simulink model "firmwareV1000_flight_replay"  (R2020b)
settings: Solver=ode1  StartTime=tspan(1)  StopTime=tspan(2)  FixedStep=Ts_SimBigModel.Ts_base  RelTol=1e-3
settings Model: PauseTimes=1  Creator=sl  LastModifiedBy=sl
settings SolverCC: AutoInsertRateTranBlk=on
settings OptimizationCC: DefaultParameterBehavior=Inlined  EnhancedBackFolding=on  PassReuseOutputArgsAs=Individual arguments  ZeroExternalMemoryAtStartup=off  ZeroInternalMemoryAtStartup=off  MaxStackSize=64  OptimizeBlockOrder=speed  DifferentSizesBufferReuse=on  OptimizationCustomize=off  EfficientTunableParamExpr=on
settings DebuggingCC: InheritedTsInSrcMsg=none  MultiTaskCondExecSysMsg=none  ParameterTunabilityLossMsg=error  UnconnectedInputMsg=none  UnconnectedOutputMsg=none  UnconnectedLineMsg=none  BusObjectLabelMismatch=error  SFUnusedDataAndEventsDiag=none
settings HardwareCC: ProdBitPerPointer=32  ProdBitPerSizeT=32  ProdBitPerPtrDiffT=32  ProdLargestAtomicInteger=Long  ProdLargestAtomicFloat=Double  ProdWordSize=32  ProdHWDeviceType=ARM Compatible->ARM Cortex
settings ModelReferenceCC: EnableParallelModelReferenceBuilds=on  ParallelModelReferenceMATLABWorkerInit=Load Top Model
settings SFSimCC: MATLABDynamicMemAlloc=off
settings RTWCC: Description=Embedded Coder  SystemTargetFile=ert.tlc  TemplateMakefile=ert_default_tmf  GenerateReport=on  Toolchain=Microsoft Visual C++ 2017 v15.0 | nmake (64-bit Windows)  IncludeHyperlinkInReport=on  LaunchReport=on  GenerateTraceInfo=on  GenerateTraceReport=on  GenerateTraceReportSl=on  GenerateTraceReportSf=on  GenerateTraceReportEml=on
settings CodeAppCC: ForceParamTrailComments=on  IgnoreCustomStorageClasses=off  OperatorAnnotations=on  SimulinkDataObjDesc=on  SFDataObjDesc=on  InsertBlockDesc=on
settings ERTTargetCC: InlinedParameterPlacement=NonHierarchical  ERTCustomFileTemplate=example_file_process.tlc

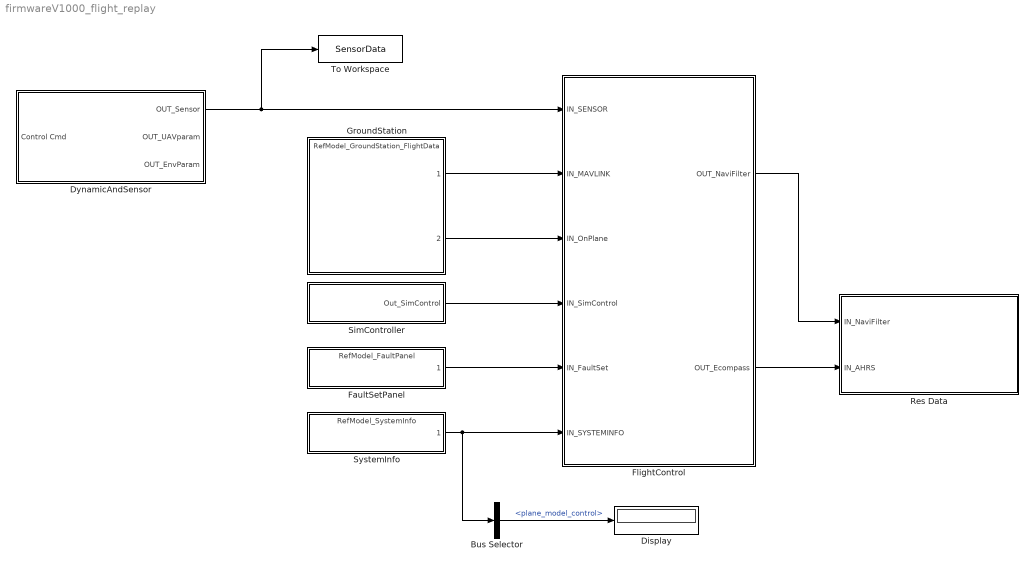
== system firmwareV1000_flight_replay ==
  Bus Selector : BusSelector  OutputSignals=plane_model_control
  Display : Display
  DynamicAndSensor : Subsystem  Variant=on
  FaultSetPanel : ModelReference  ModelNameDialog=RefModel_FaultPanel  SimulationMode=Normal  ModelReferenceVersion=2.3
  FlightControl : Subsystem
  GroundStation : ModelReference  ModelNameDialog=RefModel_GroundStation_FlightData.slx  SimulationMode=Normal  CachedPortDiscreteRates=[0.04]  ModelReferenceVersion=2.13
  Res Data : Subsystem
  SimController : Subsystem  VariantControl=SensorNoiseMode==1
  SystemInfo : ModelReference  ModelNameDialog=RefModel_SystemInfo.slx  SimulationMode=Normal  ModelReferenceVersion=2.14
  To Workspace : ToWorkspace  VariableName=SensorData  SaveFormat=Timeseries  SampleTime=-1
  wires:
  DynamicAndSensor/1(OUT_Sensor) -> FlightControl/1(IN_SENSOR), To Workspace/1
  GroundStation/2 -> FlightControl/3(IN_OnPlane)
  GroundStation/1 -> FlightControl/2(IN_MAVLINK)
  SimController/1(Out_SimControl) -> FlightControl/4(IN_SimControl)
  FaultSetPanel/1 -> FlightControl/5(IN_FaultSet)
  FlightControl/1(OUT_NaviFilter) -> Res Data/1(IN_NaviFilter)
  SystemInfo/1 -> Bus Selector/1, FlightControl/6(IN_SYSTEMINFO)
  Bus Selector/1 -> Display/1  "<plane_model_control>"
  FlightControl/2(OUT_Ecompass) -> Res Data/2(IN_AHRS)

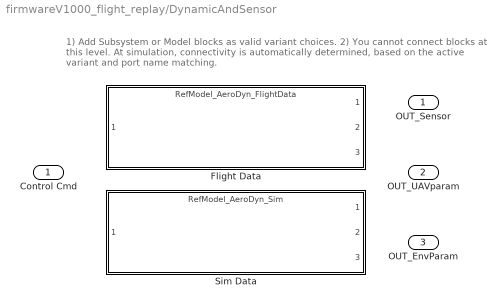
== system firmwareV1000_flight_replay/DynamicAndSensor ==
  note: 1) Add Subsystem or Model blocks as valid variant choices.
      | 2) You cannot connect blocks at this level. At simulation, connectivity is automatically
      | determined, based on the active variant and port name matching.
  Control Cmd : Inport  OutDataTypeStr=Bus: BUS_CONTROL_ACTUATOR
  Flight Data : ModelReference  DisableCoverage=on  ModelNameDialog=RefModel_AeroDyn_FlightData.slx  SimulationMode=Normal  VariantControl=SimulinkRunMode == 1  ModelReferenceVersion=2.72
  Sim Data : ModelReference  ModelNameDialog=RefModel_AeroDyn_Sim.slx  SimulationMode=Normal  VariantControl=SimulinkRunMode == 2  ModelReferenceVersion=3.4
  OUT_Sensor : Outport
  OUT_UAVparam : Outport  Port=2
  OUT_EnvParam : Outport  Port=3  LockScale=on

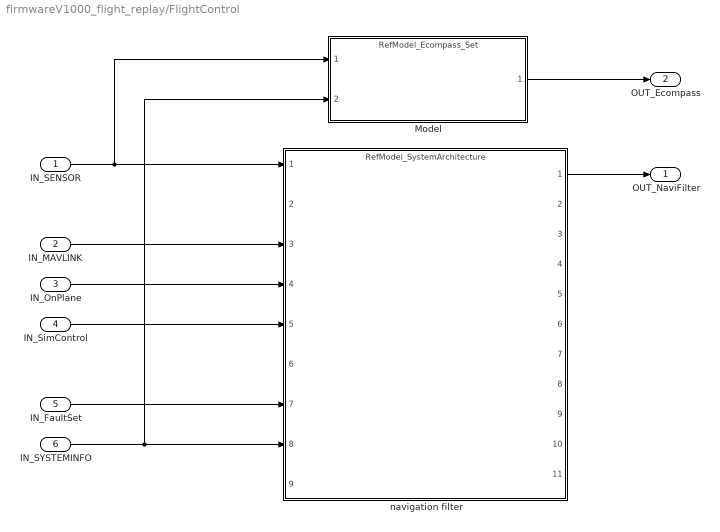
== system firmwareV1000_flight_replay/FlightControl ==
  IN_SENSOR : Inport
  IN_MAVLINK : Inport  Port=2
  IN_OnPlane : Inport  Port=3
  IN_SimControl : Inport  Port=4
  IN_FaultSet : Inport  Port=5
  IN_SYSTEMINFO : Inport  Port=6
  Model : ModelReference  ModelNameDialog=RefModel_Ecompass_Set.slx  SimulationMode=Normal  ModelReferenceVersion=2.178
  navigation filter : ModelReference  ModelNameDialog=RefModel_SystemArchitecture  SimulationMode=Normal  ModelReferenceVersion=2.174
  OUT_NaviFilter : Outport
  OUT_Ecompass : Outport  Port=2
  wires:
  IN_MAVLINK/1 -> navigation filter/3
  IN_OnPlane/1 -> navigation filter/4
  IN_SimControl/1 -> navigation filter/5
  IN_FaultSet/1 -> navigation filter/7
  navigation filter/1 -> OUT_NaviFilter/1
  IN_SENSOR/1 -> Model/1, navigation filter/1
  IN_SYSTEMINFO/1 -> Model/2, navigation filter/8
  Model/1 -> OUT_Ecompass/1

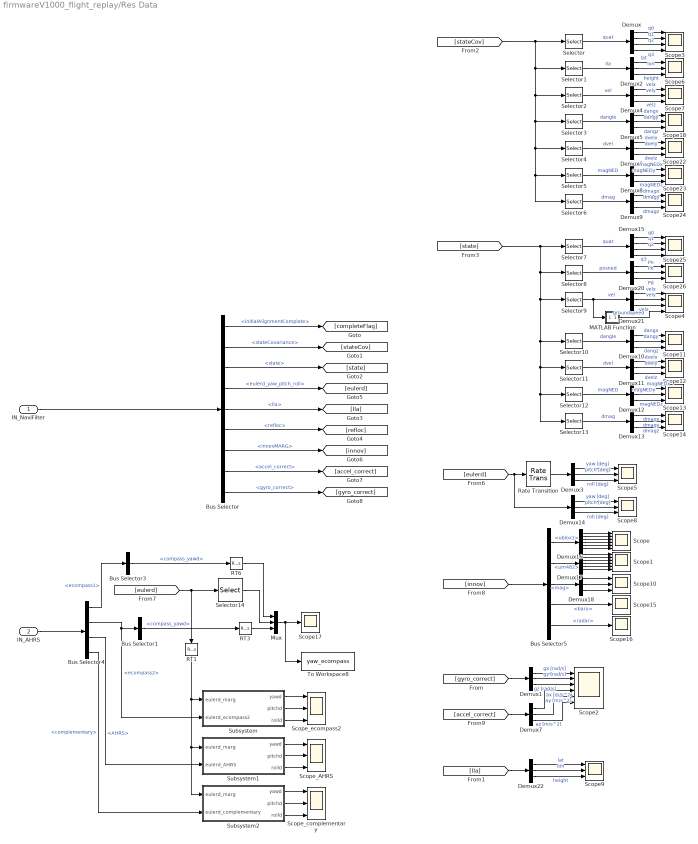
== system firmwareV1000_flight_replay/Res Data ==
  IN_NaviFilter : Inport
  IN_AHRS : Inport  Port=2
  Bus Selector : BusSelector  OutputSignals=Status.initialAlignmentComplete,stateCovariance,state,eulerd_yaw_pitch_roll,lla,InitValue.refloc,innovMARG,accel_correct,gyro_correct
  Bus Selector1 : BusSelector  OutputSignals=compass_yawd
  Bus Selector3 : BusSelector  OutputSignals=compass_yawd
  Bus Selector4 : BusSelector  OutputSignals=ecompass1,ecompass2,AHRS,complementary
  Bus Selector5 : BusSelector  OutputSignals=ublox1,um482,mag,baro,radar
  Demux : Demux
  Demux{1..14,18,20..22} (18 alike) : Demux  Outputs=3
  Demux15 : Demux
  Demux16 : Demux  Outputs=6
  Demux17 : Demux  Outputs=6
  MATLAB Function : MATLAB Function  TreatAsAtomicUnit=on
  Mux : Mux  Inputs=3
  RT1 : RateTransition
  RT3 : RateTransition
  RT6 : RateTransition
  Rate Transition : RateTransition
  Scope : Scope  NumInputPorts=6
  Scope1 : Scope  NumInputPorts=6
  Scope{5..14,18,22..24,26} (15 alike) : Scope  NumInputPorts=3
  Scope15 : Scope
  Scope16 : Scope
  Scope17 : Scope
  Scope2 : Scope  NumInputPorts=6
  Scope25 : Scope  NumInputPorts=4
  Scope3 : Scope  NumInputPorts=4
  Scope4 : Scope  NumInputPorts=4
  Scope_AHRS : Scope  NumInputPorts=3
  Scope_complementary : Scope  NumInputPorts=3
  Scope_ecompass2 : Scope  NumInputPorts=3
  Selector : Selector  InputPortWidth=NAVI_PARAM_BASE.nStateMARG24  IndexOptions=Index vector (dialog)  Indices=[1:4]  OutputSizes=1
  Selector1 : Selector  InputPortWidth=NAVI_PARAM_BASE.nStateMARG24  IndexOptions=Index vector (dialog)  Indices=[5:7]  OutputSizes=1
  Selector10 : Selector  InputPortWidth=NAVI_PARAM_BASE.nStateMARG24  IndexOptions=Index vector (dialog)  Indices=[11:13]  OutputSizes=1
  Selector11 : Selector  InputPortWidth=NAVI_PARAM_BASE.nStateMARG24  IndexOptions=Index vector (dialog)  Indices=[14:16]  OutputSizes=1
  Selector12 : Selector  InputPortWidth=NAVI_PARAM_BASE.nStateMARG24  IndexOptions=Index vector (dialog)  Indices=[17:19]  OutputSizes=1
  Selector13 : Selector  InputPortWidth=NAVI_PARAM_BASE.nStateMARG24  IndexOptions=Index vector (dialog)  Indices=[20:22]  OutputSizes=1
  Selector14 : Selector  InputPortWidth=3  IndexOptions=Index vector (dialog)  Indices=1  OutputSizes=1
  Selector2 : Selector  InputPortWidth=NAVI_PARAM_BASE.nStateMARG24  IndexOptions=Index vector (dialog)  Indices=[8:10]  OutputSizes=1
  Selector3 : Selector  InputPortWidth=NAVI_PARAM_BASE.nStateMARG24  IndexOptions=Index vector (dialog)  Indices=[11:13]  OutputSizes=1
  Selector4 : Selector  InputPortWidth=NAVI_PARAM_BASE.nStateMARG24  IndexOptions=Index vector (dialog)  Indices=[14:16]  OutputSizes=1
  Selector5 : Selector  InputPortWidth=NAVI_PARAM_BASE.nStateMARG24  IndexOptions=Index vector (dialog)  Indices=[17:19]  OutputSizes=1
  Selector6 : Selector  InputPortWidth=NAVI_PARAM_BASE.nStateMARG24  IndexOptions=Index vector (dialog)  Indices=[20:22]  OutputSizes=1
  Selector7 : Selector  InputPortWidth=NAVI_PARAM_BASE.nStateMARG24  IndexOptions=Index vector (dialog)  Indices=[1:4]  OutputSizes=1
  Selector8 : Selector  InputPortWidth=NAVI_PARAM_BASE.nStateMARG24  IndexOptions=Index vector (dialog)  Indices=[5:7]  OutputSizes=1
  Selector9 : Selector  InputPortWidth=NAVI_PARAM_BASE.nStateMARG24  IndexOptions=Index vector (dialog)  Indices=[8:10]  OutputSizes=1
  Subsystem : Subsystem
  Subsystem1 : Subsystem
  Subsystem2 : Subsystem
  To Workspace8 : ToWorkspace  VariableName=yaw_ecompass  SaveFormat=Timeseries  SampleTime=-1
  wires:
  Demux13/1 -> Scope14/1  "dmagx"
  Demux12/2 -> Scope13/2  "magNEDy"
  Demux12/1 -> Scope13/1  "magNEDx"
  Demux3/2 -> Scope5/2  "pitch [deg]"
  Selector10/1 -> Demux10/1  "dangle"
  Demux21/3 -> Scope4/3  "velz"
  Selector14/1 -> Mux/2
  Demux/2 -> Scope3/2  "q1"
  [eulerd] -> Selector14/1, RT1/1
  [state] -> Selector8/1, Selector11/1, Selector12/1, Selector13/1, Selector10/1, Selector9/1, Selector7/1
  Demux6/3 -> Scope22/3  "dvelz"
  Demux5/2 -> Scope18/2  "dangy"
  Demux11/1 -> Scope12/1  "dvelx"
  Bus Selector1/1 -> RT3/1  "<compass_yawd>"
  Subsystem/3(rolld) -> Scope_ecompass2/3
  Demux16/3 -> Scope/3
  Demux3/1 -> Scope5/1  "yaw [deg]"
  Bus Selector5/5 -> Scope16/1  "<radar>"
  Demux17/1 -> Scope1/1
  Bus Selector4/1 -> Bus Selector3/1  "<ecompass1>"
  Bus Selector5/4 -> Scope15/1  "<baro>"
  Demux/1 -> Scope3/1  "q0"
  Demux6/2 -> Scope22/2  "dvely"
  Demux9/1 -> Scope24/1  "dmagx"
  Bus Selector/9 -> [gyro_correct]  "<gyro_correct>"
  Bus Selector5/2 -> Demux17/1  "<um482>"
  Demux2/3 -> Scope6/3  "height"
  Demux14/3 -> Scope8/3  "roll [deg]"
  RT1/1 -> Subsystem2/1(eulerd_marg), Subsystem1/1(eulerd_marg), Subsystem/1(eulerd_marg)
  Selector1/1 -> Demux2/1  "lla"
  Demux18/1 -> Scope10/1
  Demux21/2 -> Scope4/2  "vely"
  Bus Selector4/4 -> Subsystem2/2(eulerd_complementary)  "<complementary>"
  Bus Selector5/3 -> Demux18/1  "<mag>"
  Demux17/2 -> Scope1/2
  [lla] -> Demux22/1
  Rate Transition/1 -> Demux3/1
  Bus Selector/4 -> [eulerd]  "<eulerd_yaw_pitch_roll>"
  Subsystem1/1(yawd) -> Scope_AHRS/1
  Demux6/1 -> Scope22/1  "dvelx"
  Demux17/4 -> Scope1/4
  Demux17/3 -> Scope1/3
  Demux11/2 -> Scope12/2  "dvely"
  Bus Selector5/1 -> Demux16/1  "<ublox1>"
  Demux16/1 -> Scope/1
  MATLAB Function/1(y) -> Scope4/4  "groundspeed"
  Demux20/1 -> Scope26/1  "Pn"
  Demux17/6 -> Scope1/6
  Demux16/4 -> Scope/4
  Demux15/2 -> Scope25/2  "q1"
  Demux16/5 -> Scope/5
  Bus Selector4/2 -> Subsystem/2(eulerd_ecompass2), Bus Selector1/1  "<ecompass2>"
  Demux17/5 -> Scope1/5
  Bus Selector/2 -> [stateCov]  "<stateCovariance>"
  Demux10/1 -> Scope11/1  "dangx"
  Selector12/1 -> Demux12/1  "magNED"
  IN_NaviFilter/1 -> Bus Selector/1
  Demux4/3 -> Scope7/3  "velz"
  Mux/1 -> To Workspace8/1, Scope17/1
  [eulerd] -> Demux14/1, Rate Transition/1
  Subsystem/2(pitchd) -> Scope_ecompass2/2
  Bus Selector/5 -> [lla]  "<lla>"
  Subsystem1/3(rolld) -> Scope_AHRS/3
  Demux14/1 -> Scope8/1  "yaw [deg]"
  Subsystem2/3(rolld) -> Scope_complementary/3
  Subsystem2/1(yawd) -> Scope_complementary/1
  Selector2/1 -> Demux4/1  "vel"
  Demux3/3 -> Scope5/3  "roll [deg]"
  Subsystem2/2(pitchd) -> Scope_complementary/2
  Subsystem/1(yawd) -> Scope_ecompass2/1
  Demux1/2 -> Scope2/2  "gy [rad/s]"
  Demux22/3 -> Scope9/3  "height"
  Demux22/1 -> Scope9/1  "lat"
  Demux15/3 -> Scope25/3  "q2"
  Demux1/3 -> Scope2/3  "gz [rad/s]"
  Selector5/1 -> Demux8/1  "magNED"
  Bus Selector3/1 -> RT6/1  "<compass_yawd>"
  Demux7/1 -> Scope2/4  "ax [m/s^2]"
  Demux1/1 -> Scope2/1  "gx [rad/s]"
  Bus Selector/7 -> [innov]  "<innovMARG>"
  Demux14/2 -> Scope8/2  "pitch [deg]"
  [innov] -> Bus Selector5/1
  [accel_correct] -> Demux7/1
  Demux7/3 -> Scope2/6  "az [m/s^2]"
  Bus Selector/3 -> [state]  "<state>"
  Demux11/3 -> Scope12/3  "dvelz"
  Demux5/3 -> Scope18/3  "dangz"
  Bus Selector/1 -> [completeFlag]  "<initialAlignmentComplete>"
  Bus Selector/8 -> [accel_correct]  "<accel_correct>"
  Bus Selector/6 -> [refloc]  "<refloc>"
  Demux20/3 -> Scope26/3  "Pd"
  Demux8/3 -> Scope23/3  "magNEDz"
  Demux4/1 -> Scope7/1  "velx"
  Demux5/1 -> Scope18/1  "dangx"
  Selector4/1 -> Demux6/1  "dvel"
  Demux9/2 -> Scope24/2  "dmagy"
  Demux10/2 -> Scope11/2  "dangy"
  [gyro_correct] -> Demux1/1
  Demux2/2 -> Scope6/2  "lon"
  Demux10/3 -> Scope11/3  "dangz"
  Demux16/2 -> Scope/2
  Selector11/1 -> Demux11/1  "dvel"
  Demux13/3 -> Scope14/3  "dmagz"
  Demux18/2 -> Scope10/2
  Selector8/1 -> Demux20/1  "posned"
  Demux4/2 -> Scope7/2  "vely"
  Demux13/2 -> Scope14/2  "dmagy"
  Selector9/1 -> MATLAB Function/1(vel), Demux21/1  "vel"
  Subsystem1/2(pitchd) -> Scope_AHRS/2
  Demux12/3 -> Scope13/3  "magNEDz"
  Selector7/1 -> Demux15/1  "quat"
  Demux8/2 -> Scope23/2  "magNEDy"
  Demux/3 -> Scope3/3  "q2"
  Demux15/4 -> Scope25/4  "q3"
  Bus Selector4/3 -> Subsystem1/2(eulerd_AHRS)  "<AHRS>"
  IN_AHRS/1 -> Bus Selector4/1
  Selector13/1 -> Demux13/1  "dmag"
  Demux8/1 -> Scope23/1  "magNEDx"
  Demux21/1 -> Scope4/1  "velx"
  Demux9/3 -> Scope24/3  "dmagz"
  Selector3/1 -> Demux5/1  "dangle"
  Demux18/3 -> Scope10/3
  Demux/4 -> Scope3/4  "q3"
  RT3/1 -> Mux/3
  Selector6/1 -> Demux9/1  "dmag"
  Demux20/2 -> Scope26/2  "Pe"
  Demux7/2 -> Scope2/5  "ay [m/s^2]"
  Demux22/2 -> Scope9/2  "lon"
  Demux15/1 -> Scope25/1  "q0"
  [stateCov] -> Selector/1, Selector3/1, Selector4/1, Selector5/1, Selector6/1, Selector2/1, Selector1/1
  Demux2/1 -> Scope6/1  "lat"
  Demux16/6 -> Scope/6
  Selector/1 -> Demux/1  "quat"
  RT6/1 -> Mux/1

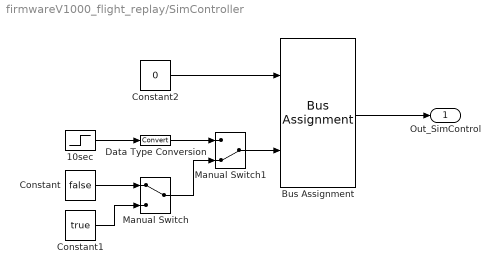
== system firmwareV1000_flight_replay/SimController ==
  10sec : Step  Time=10+33  mask(DiscretizedSource){}
      mask init:
      | %zoh
  Bus Assignment : BusAssignment  AssignedSignals=isSimOn
  Constant : Constant  Value=false
  Constant1 : Constant  Value=true
  Constant2 : Constant  Value=0  OutDataTypeStr=Bus: BUS_SIMCONTROL
  Data Type Conversion : DataTypeConversion
  Manual Switch : ManualSwitch
  Manual Switch1 : ManualSwitch  CurrentSetting=0
  Out_SimControl : Outport
  wires:
  Constant/1 -> Manual Switch/1
  Constant1/1 -> Manual Switch/2
  Constant2/1 -> Bus Assignment/1
  Bus Assignment/1 -> Out_SimControl/1
  Manual Switch1/1 -> Bus Assignment/2
  Manual Switch/1 -> Manual Switch1/2
  10sec/1 -> Data Type Conversion/1
  Data Type Conversion/1 -> Manual Switch1/1

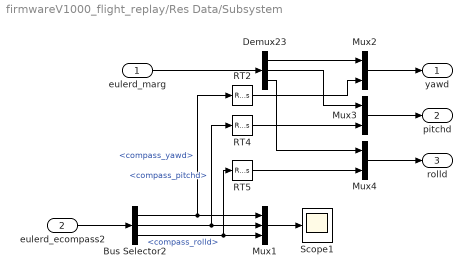
== system firmwareV1000_flight_replay/Res Data/Subsystem ==
  eulerd_marg : Inport
  eulerd_ecompass2 : Inport  Port=2
  Bus Selector2 : BusSelector  OutputSignals=compass_yawd,compass_pitchd,compass_rolld
  Demux23 : Demux  Outputs=3
  Mux1 : Mux  Inputs=3
  Mux2 : Mux  Inputs=2
  Mux3 : Mux  Inputs=2
  Mux4 : Mux  Inputs=2
  RT2 : RateTransition
  RT4 : RateTransition
  RT5 : RateTransition
  Scope1 : Scope
  yawd : Outport
  pitchd : Outport  Port=2
  rolld : Outport  Port=3
  wires:
  RT4/1 -> Mux3/2
  Demux23/1 -> Mux2/1
  RT2/1 -> Mux2/2
  Mux1/1 -> Scope1/1
  Bus Selector2/2 -> RT4/1, Mux1/2  "<compass_pitchd>"
  Demux23/3 -> Mux4/1
  eulerd_marg/1 -> Demux23/1
  Bus Selector2/3 -> RT5/1, Mux1/3  "<compass_rolld>"
  RT5/1 -> Mux4/2
  Demux23/2 -> Mux3/1
  Bus Selector2/1 -> Mux1/1, RT2/1  "<compass_yawd>"
  Mux4/1 -> rolld/1
  eulerd_ecompass2/1 -> Bus Selector2/1
  Mux3/1 -> pitchd/1
  Mux2/1 -> yawd/1

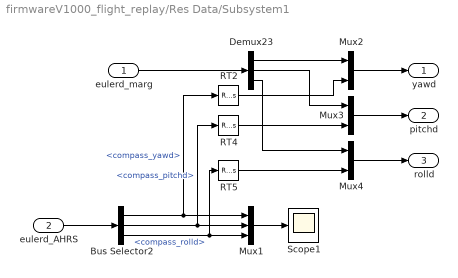
== system firmwareV1000_flight_replay/Res Data/Subsystem1 ==
  eulerd_marg : Inport
  eulerd_AHRS : Inport  Port=2
  Bus Selector2 : BusSelector  OutputSignals=compass_yawd,compass_pitchd,compass_rolld
  Demux23 : Demux  Outputs=3
  Mux1 : Mux  Inputs=3
  Mux2 : Mux  Inputs=2
  Mux3 : Mux  Inputs=2
  Mux4 : Mux  Inputs=2
  RT2 : RateTransition
  RT4 : RateTransition
  RT5 : RateTransition
  Scope1 : Scope
  yawd : Outport
  pitchd : Outport  Port=2
  rolld : Outport  Port=3
  wires:
  Mux2/1 -> yawd/1
  Mux3/1 -> pitchd/1
  eulerd_AHRS/1 -> Bus Selector2/1
  Mux4/1 -> rolld/1
  Bus Selector2/1 -> RT2/1, Mux1/1  "<compass_yawd>"
  Demux23/2 -> Mux3/1
  RT5/1 -> Mux4/2
  Bus Selector2/3 -> Mux1/3, RT5/1  "<compass_rolld>"
  eulerd_marg/1 -> Demux23/1
  Demux23/3 -> Mux4/1
  Bus Selector2/2 -> Mux1/2, RT4/1  "<compass_pitchd>"
  Mux1/1 -> Scope1/1
  RT2/1 -> Mux2/2
  Demux23/1 -> Mux2/1
  RT4/1 -> Mux3/2

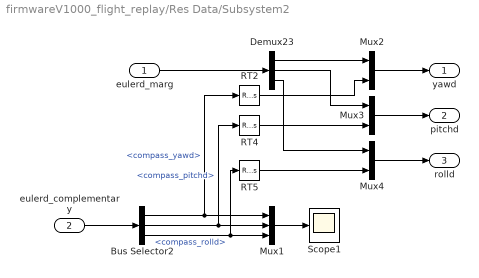
== system firmwareV1000_flight_replay/Res Data/Subsystem2 ==
  eulerd_marg : Inport
  eulerd_complementary : Inport  Port=2
  Bus Selector2 : BusSelector  OutputSignals=compass_yawd,compass_pitchd,compass_rolld
  Demux23 : Demux  Outputs=3
  Mux1 : Mux  Inputs=3
  Mux2 : Mux  Inputs=2
  Mux3 : Mux  Inputs=2
  Mux4 : Mux  Inputs=2
  RT2 : RateTransition
  RT4 : RateTransition
  RT5 : RateTransition
  Scope1 : Scope
  yawd : Outport
  pitchd : Outport  Port=2
  rolld : Outport  Port=3
  wires:
  RT4/1 -> Mux3/2
  Demux23/1 -> Mux2/1
  RT2/1 -> Mux2/2
  Mux1/1 -> Scope1/1
  Bus Selector2/2 -> RT4/1, Mux1/2  "<compass_pitchd>"
  Demux23/3 -> Mux4/1
  eulerd_marg/1 -> Demux23/1
  Bus Selector2/3 -> RT5/1, Mux1/3  "<compass_rolld>"
  RT5/1 -> Mux4/2
  Demux23/2 -> Mux3/1
  Bus Selector2/1 -> Mux1/1, RT2/1  "<compass_yawd>"
  Mux4/1 -> rolld/1
  eulerd_complementary/1 -> Bus Selector2/1
  Mux3/1 -> pitchd/1
  Mux2/1 -> yawd/1

== matlab function firmwareV1000_flight_replay/Res Data/MATLAB Function ==
  data: vel input; y output
function y = fcn(vel)

y = norm(vel(1:2));
